simulink library "monroe_library"  (R2012b)
settings: Solver=ode45  StartTime=0.0  StopTime=10.0  RelTol=1e-3
values from neighbouring files (symbols this model uses):
  input_bit_width = ', num2str(input_bit_width))    [fft_direct_draw.m]
undefined symbols (not defined in the file or in its folder): gcbh, xlBlockLoadCallback
libraries: xbsIndex_r4 x1880, monroe_library x159, casper_library x13, xps_library x1
(part 17 of 43)

== system monroe_library/direct_coeff_gen/coeff_gen_stage_1_group_4 ==
  sync : Inport
  Concat : xbsIndex_r4/Concat  num_inputs=2  dbl_ovrd=off  block_type=concat
  Concat1 : xbsIndex_r4/Concat  num_inputs=2  dbl_ovrd=off  block_type=concat
  Concat2 : xbsIndex_r4/Concat  num_inputs=2  dbl_ovrd=off  block_type=concat
  Constant : xbsIndex_r4/Constant  arith_type=Boolean  const=0  n_bits=16  bin_pt=14  explicit_period=on  period=1  equ=P=C  opselect=C  inp2=PCIN>>17  opr=+  inp1=P  carry=CIN  dbl_ovrd=off  block_type=constant
  Constant1 : xbsIndex_r4/Constant  arith_type=Boolean  const=1  n_bits=16  bin_pt=14  explicit_period=off  period=1  equ=P=C  opselect=C  inp2=PCIN>>17  opr=+  inp1=P  carry=CIN  dbl_ovrd=off  block_type=constant
  Constant3 : xbsIndex_r4/Constant  arith_type=Signed (2's comp)  const=0  n_bits=18  bin_pt=17  explicit_period=on  period=1  equ=P=C  opselect=C  inp2=PCIN>>17  opr=+  inp1=P  carry=CIN  dbl_ovrd=off  block_type=constant
  Constant4 : xbsIndex_r4/Constant  arith_type=Boolean  const=0  n_bits=16  bin_pt=14  explicit_period=off  period=1  equ=P=C  opselect=C  inp2=PCIN>>17  opr=+  inp1=P  carry=CIN  dbl_ovrd=off  block_type=constant
  Constant5 : xbsIndex_r4/Constant  arith_type=Unsigned  const=2  n_bits=10  bin_pt=0  explicit_period=on  period=1  equ=P=C  opselect=C  inp2=PCIN>>17  opr=+  inp1=P  carry=CIN  dbl_ovrd=off  block_type=constant
  Counter : xbsIndex_r4/Counter  cnt_type=Free Running  cnt_to=Inf  operation=Up  start_count=0  cnt_by_val=1  arith_type=Unsigned  n_bits=10  bin_pt=0  load_pin=on  rst=off  en=off  explicit_period=on  period=1  dbl_ovrd=off  use_behavioral_HDL=off  implementation=Fabric  block_type=counter
  Delay : xbsIndex_r4/Delay  en=off  latency=0  dbl_ovrd=off  reg_retiming=off  block_type=delay
  Dual Port RAM4 : xbsIndex_r4/Dual Port RAM  depth=2048  initVector=[0 -0.00306795676296598 -0.00613588464915448 -0.00920375478205982 -0.0122715382857199 -0.0153392062849881 -0.0184067299058048 -0.0214740802754695 -0.0245412285229123 -0.0276081457789657 -0.0306748031766366 -0.0337411718513776 -0.0368072229413588 -0.0398729275877398 -0.0429382569349408 -0.0460031821309146 -0.049067674327418 -0.0521317046802833 -0.0551952443496899 -0.0582582645004358 -0.0613207363022086 -0.0643826309298575 -0.0674439195636641 -0.0705045733896139 -0.0735645635996674 -0.0766238613920315 -0.0796824379714301 -0.0827402645493757 -0.0857973123444399 -0.0888535525825246 -0.0919089564971327 -0.094963495329639 -0.0980171403295606 -0.101069862754828 -0.104121633872055 -0.107172424956809 -0.110222207293883 -0.113270952177564 -0.116318630911905 -0.119365214810991 -0.122410675199216 -0.125454983411546 -0.128498110793793 -0.131540028702883 -0.134580708507126 -0.137620121586486 -0.140658239332849 -0.143695033150294 -0.146730474455362 -0.149764534677322 -0.152797185258443 -0.155828397654265 -0.158858143333861 -0.161886393780112 -0.16491312048997 -0.167938294974731 -0.170961888760301 -0.173983873387464 -0.177004220412149 -0.1800229014057 -0.183039887955141 -0.186055151663447 -0.189068664149806 -0.192080397049892 -0.195090322016128 -0.198098410717954 -0.201104634842092 -0.204108966092817 -0.207111376192219 -0.21011183688047 -0.213110319916091 -0.21610679707622 -0.21910124015687 -0.222093620973204 -0.225083911359793 -0.228072083170886 -0.231058108280671 -0.234041958583543 -0.237023605994367 -0.240003022448741 -0.242980179903264 -0.245955050335795 -0.24892760574572 -0.251897818154217 -0.254865659604515 -0.257831102162159 -0.260794117915276 -0.263754678974831 -0.266712757474898 -0.269668325572915 -0.272621355449949 -0.275571819310958 -0.278519689385053 -0.281464937925758 -0.284407537211272 -0.28734745954473 -0.290284677254462 -0.293219162694259 -0.296150888243624 -0.29907982630804 -0.302005949319228 -0.304929229735402 -0.307849640041535 -0.310767152749611 -0.313681740398892 -0.316593375556166 -0.319502030816016 -0.32240767880107 -0.325310292162263 -0.328209843579092 -0.331106305759876 -0.333999651442009 -0.33688985339222 -0.339776884406827 -0.342660717311994 -0.345541324963989 -0.348418680249435 -0.351292756085567 -0.35416352542049 -0.35703096123343 -0.359895036534988 -0.362755724367397 -0.365612997804774 -0.368466829953372 -0.371317193951837 -0.374164062971458 -0.377007410216418 -0.379847208924051 -0.38268343236509 -0.385516053843919 -0.388345046698826 -0.391170384302254 -0.393992040061048 -0.39680998741671 -0.399624199845647 -0.402434650859418 -0.40524131400499 -0.408044162864979 -0.410843171057904 -0.413638312238435 -0.416429560097637 -0.419216888363224 -0.4220002707998 -0.424779681209109 -0.427555093430282 -0.430326481340083 -0.433093818853152 -0.435857079922255 -0.438616238538528 -0.441371268731717 -0.444122144570429 -0.446868840162374 -0.449611329654607 -0.452349587233771 -0.455083587126344 -0.457813303598877 -0.46053871095824 -0.46325978355186 -0.465976495767966 -0.468688822035828 -0.471396736825998 -0.47410021465055 -0.476799230063322 -0.479493757660153 -0.482183772079123 -0.484869248000791 -0.487550160148436 -0.490226483288291 -0.492898192229784 -0.495565261825773 -0.498227666972782 -0.500885382611241 -0.503538383725718 -0.506186645345155 -0.508830142543107 -0.51146885043797 -0.514102744193222 -0.51673179901765 -0.51935599016559 -0.521975292937154 -0.524589682678469 -0.527199134781901 -0.529803624686295 -0.532403127877198 -0.534997619887097 -0.537587076295645 -0.540171472729893 -0.542750784864516 -0.545324988422046 -0.5478940591731 -0.550457972936605 -0.553016705580027 -0.555570233019602 -0.558118531220556 -0.560661576197336 -0.563199344013834 -0.565731810783613 -0.568258952670131 -0.570780745886967 -0.573297166698042 -0.575808191417845 -0.578313796411656 -0.580813958095765 -0.583308652937698 -0.585797857456439 -0.588281548222645 -0.590759701858874 -0.5932322950398 -0.595699304492433 -0.598160706996342 -0.600616479383869 ...(+34229 chars)]  distributed_mem=Block RAM  init_a=0  init_b=0  rst_a=off  rst_b=off  en_a=off  en_b=off  latency=2  write_mode_A=No Read On Write  write_mode_B=No Read On Write  dbl_ovrd=off  optimize=Area  use_rpm=on  block_type=dpram
  Reinterpret : xbsIndex_r4/Reinterpret  force_arith_type=on  arith_type=Unsigned  force_bin_pt=on  bin_pt=0  block_type=reinterpret
      settings: infoedit="Changes signal type without altering the binary representation.   You can changed the signal between signed and unsigned, and relocate the binary point.<br><br>Hardware notes: In hardware this block costs nothing.<br><br>Example:  Suppose the input is 6 bits wide, signed, with 2 fractional bits, and the output is forced to unsigned with 0 fractional bits.  Then an input of -2.0 (1110.00 in binary 2's complement) becomes an output of 56 (111000 in binary)."
  Reinterpret1 : xbsIndex_r4/Reinterpret  force_arith_type=on  arith_type=Unsigned  force_bin_pt=on  bin_pt=0  block_type=reinterpret
      settings: infoedit="Changes signal type without altering the binary representation.   You can changed the signal between signed and unsigned, and relocate the binary point.<br><br>Hardware notes: In hardware this block costs nothing.<br><br>Example:  Suppose the input is 6 bits wide, signed, with 2 fractional bits, and the output is forced to unsigned with 0 fractional bits.  Then an input of -2.0 (1110.00 in binary 2's complement) becomes an output of 56 (111000 in binary)."
  count_slice : xbsIndex_r4/Slice  nbits=10  boolean_output=off  mode=Upper Bit Location + Width  bit1=0  base1=MSB of Input  bit0=0  base0=MSB of Input  dbl_ovrd=off  block_type=slice
  coeff : Outport
  wires:
  count_slice/1 -> Concat1/2, Concat/2  "xlsub2_Counter_out1"
  Constant3/1 -> Dual Port RAM4/5, Dual Port RAM4/2  "xlsub2_Constant3_out1"
  Constant/1 -> Dual Port RAM4/6, Dual Port RAM4/3  "xlsub2_Constant_out1"
  Reinterpret1/1 -> Concat2/2  "xlsub2_Reinterpret1_out1"
  Dual Port RAM4/2 -> Reinterpret1/1  "xlsub2_Dual_Port_RAM4_out2"
  Reinterpret/1 -> Concat2/1  "xlsub2_Reinterpret_out1"
  Dual Port RAM4/1 -> Reinterpret/1  "xlsub2_Dual_Port_RAM4_out1"
  Concat1/1 -> Dual Port RAM4/4  "xlsub2_Concat1_out1"
  Concat/1 -> Dual Port RAM4/1  "xlsub2_Concat_out1"
  Delay/1 -> coeff/1
  Concat2/1 -> Delay/1  "xlsub2_Concat2_out1"
  Counter/1 -> count_slice/1
  Constant5/1 -> Counter/2  "xlsub2_Constant5_out1"
  sync/1 -> Counter/1
  Constant4/1 -> Concat1/1  "xlsub2_Constant4_out1"
  Constant1/1 -> Concat/1  "xlsub2_Constant1_out1"
